simulink model "Control_model_10DOF_fin"  (R2016b)
settings: Solver=FixedStepAuto  StartTime=0.0  StopTime=10  FixedStep=0.0001  RelTol=1e-3
InitFcn:
  | Initialisation_ctr_10DOF_fin
values from neighbouring files (symbols this model uses):
  COM_Parameters = [-lpelvis/2;r2;0]    [Initialisation_ctr_10DOF_fin.m]
  DH_Parameters = [hfoot 0 ... (first row only)    [Initialisation_ctr_10DOF_fin.m]
  dTrunk = trunklbd(3)    [Initialisation_ctr_10DOF_fin.m]
  dxFootSM = dxFoot    [Initialisation_ctr_10DOF_fin.m]
  dxTrunk = 0.1    [Initialisation_ctr_10DOF_fin.m]
  Foot_Parameters = [0;-(lFoot/2-lHeel);0]    [Initialisation_ctr_10DOF_fin.m]
  HAA2HEE = [0; 0; 0.001]    [Initialisation_ctr_10DOF_fin.m]
  HEE2HFE = 0.5*[0.2; 0; 0]    [Initialisation_ctr_10DOF_fin.m]
  height_vrp = CoM_position(1)    [Initialisation_ctr_10DOF_fin.m]
  hTrunk = trunklbd(1)    [Initialisation_ctr_10DOF_fin.m]
  initial_CoM_position = R*CoM_position    [Initialisation_ctr_10DOF_fin.m]
  initial_CoM_velocity = [0;0;0]    [Initialisation_ctr_10DOF_fin.m]
  initial_left_foot = [0;0;-stance_width/2]    [Initialisation_ctr_10DOF_fin.m]
  initial_right_foot = [0;0;stance_width/2]    [Initialisation_ctr_10DOF_fin.m]
  initial_RorL = 0    [Initialisation_ctr_10DOF_fin.m]
  jointsinitial = [9;-15;6;0;0;6;-15;9]/180*pi    [Initialisation_ctr_10DOF_fin.m]
  K_DCM = 4.3*[1 0 0 ... (first row only)    [Initialisation_ctr_10DOF_fin.m]
  kD_left = mbody*[0.95 0 0 0 ... (first row only)    [Initialisation_ctr_10DOF_fin.m]
  kD_right = mbody*[0.12 0 0 0 ... (first row only)    [Initialisation_ctr_10DOF_fin.m]
  kI_left = mbody*[35 0 0 0 ... (first row only)    [Initialisation_ctr_10DOF_fin.m]
  kI_right = mbody*[38.2 0 0 0 ... (first row only)    [Initialisation_ctr_10DOF_fin.m]
  kP_left = mbody*[75 0 0 0 ... (first row only)    [Initialisation_ctr_10DOF_fin.m]
  kP_right = mbody*[5.6 0 0 0 ... (first row only)    [Initialisation_ctr_10DOF_fin.m]
  Lenght = [lShank;lThigh]    [Initialisation_ctr_10DOF_fin.m]
  lFootSM = lFoot    [Initialisation_ctr_10DOF_fin.m]
  lpelvis = wPelvis    [Initialisation_ctr_10DOF_fin.m]
  mass = mbody    (= 60)    [Initialisation_ctr_10DOF_fin.m]
  Masses = [mThigh; mShank; mTrunk]    [Initialisation_ctr_10DOF_fin.m]
  nb_step = 4    [Initialisation_ctr_10DOF_fin.m]
  nb_step_pattern = 20    [Initialisation_ctr_10DOF_fin.m]
  Pelvis_Parameters = [-lpelvis/2;hTrunk/2;0]    [Initialisation_ctr_10DOF_fin.m]
  stance_width = lpelvis    [Initialisation_ctr_10DOF_fin.m]
  stride_lenght = 0.50    (= 0.5)    [Initialisation_ctr_10DOF_fin.m]
  T_DS = time_DS    (= 0.4)    [Initialisation_ctr_10DOF_fin.m]
  T_IT = time_DS    (= 0.4)    [Initialisation_ctr_10DOF_fin.m]
  T_SS = time_swing    (= 1.6)    [Initialisation_ctr_10DOF_fin.m]
  time_DS = (time_stance-time_swing)/2    (= 0.4)    [Initialisation_ctr_10DOF_fin.m]
  time_stance = 60/100*time_stride    (= 2.4)    [Initialisation_ctr_10DOF_fin.m]
  time_step = time_stride/2    (= 2)    [Initialisation_ctr_10DOF_fin.m]
  time_swing = 40/100*time_stride    (= 1.6)    [Initialisation_ctr_10DOF_fin.m]
  validity_angle = [-20*pi/180 20*pi/180 ... (first row only)    [Initialisation_ctr_10DOF_fin.m]
  wTrunk = trunklbd(2)    [Initialisation_ctr_10DOF_fin.m]
  x4CoM = CoM_position(1)-XR4(1)    [Initialisation_ctr_10DOF_fin.m]
undefined symbols (not defined in the file or in its folder): dsegment, hFoot, l, lFoot, omega0_x, omega0_z, rho, wPelvis, X, Xp_x, Xp_z, Y, Z
undefined symbols (not defined in the file): k_grf, lShankSM, lThighSM, mShank, mThigh
libraries: nesl_utility x247, sm_lib x215, dspindex x12, FootPlacementLibrary x8, dspsigops x4, dspswit3 x1
(part 10 of 18)

== system Control_model_10DOF_fin/10DoF Walker SimMechanics Model/Graphic/Subsystem/Subsystem6 ==
  In1 : Inport
  Cartesian Joint : sm_lib/Joints/Cartesian Joint  SenseConstraintForce=off  SenseConstraintForceX=off  SenseConstraintForceY=off  SenseConstraintForceZ=off  SenseConstraintTorque=off  SenseConstraintTorqueX=off  SenseConstraintTorqueY=off  SenseConstraintTorqueZ=off  SenseTotalForce=off  SenseTotalForceX=off  SenseTotalForceY=off  SenseTotalForceZ=off  SenseTotalTorque=off  SenseTotalTorqueX=off  SenseTotalTorqueY=off  SenseTotalTorqueZ=off  CompositeWrenchDir=FollowerOnBase  CompositeWrenchFrame=BaseFrame  PxEquilibriumPosition=0  PxEquilibriumPositionUnits=m  PxSpringStiffness=0  PxSpringStiffnessUnits=N/m  PxDampingCoefficient=0  PxDampingCoefficientUnits=N/(m/s)  PxTorqueActuationMode=ComputedTorque  PxMotionActuationMode=InputMotion  PxSensePosition=off  PxSenseVelocity=off  PxSenseAcceleration=off  PxSenseTorqueForce=off  PxPositionTargetSpecify=on  PxPositionTargetPriority=Low  PxPositionTargetValue=0  PxPositionTargetValueUnits=m  PxVelocityTargetSpecify=off  PxVelocityTargetPriority=High  PxVelocityTargetValue=0  PxVelocityTargetValueUnits=m/s  PyEquilibriumPosition=0  PyEquilibriumPositionUnits=m  PySpringStiffness=0  PySpringStiffnessUnits=N/m  PyDampingCoefficient=0  PyDampingCoefficientUnits=N/(m/s)  PyTorqueActuationMode=ComputedTorque  PyMotionActuationMode=InputMotion  PySensePosition=off  PySenseVelocity=off  PySenseAcceleration=off  PySenseTorqueForce=off  PyPositionTargetSpecify=on  PyPositionTargetPriority=Low  PyPositionTargetValue=0  PyPositionTargetValueUnits=m  PyVelocityTargetSpecify=off  PyVelocityTargetPriority=High  PyVelocityTargetValue=0  PyVelocityTargetValueUnits=m/s  PzEquilibriumPosition=0  PzEquilibriumPositionUnits=m  PzSpringStiffness=0  PzSpringStiffnessUnits=N/m  PzDampingCoefficient=0  PzDampingCoefficientUnits=N/(m/s)  PzTorqueActuationMode=ComputedTorque  PzMotionActuationMode=InputMotion  PzSensePosition=off  PzSenseVelocity=off  PzSenseAcceleration=off  PzSenseTorqueForce=off  PzPositionTargetSpecify=on  PzPositionTargetPriority=Low  PzPositionTargetValue=0  PzPositionTargetValueUnits=m  PzVelocityTargetSpecify=off  PzVelocityTargetPriority=High  PzVelocityTargetValue=0  PzVelocityTargetValueUnits=m/s
  Demux : Demux  Outputs=3
  Graphic : sm_lib/Body Elements/Graphic  GraphicType=Marker  MarkerShape=Sphere  MarkerSize=10  GraphicVisPropType=SimpleVisualProperties  GraphicDiffuseColor=[0.2 0.2 1.0]  GraphicSpecularColor=[0.5 0.5 0.5 1.0]  GraphicAmbientColor=[0.15 0.15 0.15 1.0]  GraphicEmissiveColor=[0.0 0.0 0.0 1.0]  GraphicShininess=75  GraphicOpacity=1.0
  Memory2 : Memory  X0=[0;0;0]
  Rigid Transform1 : sm_lib/Frames and Transforms/Rigid Transform  TranslationMethod=None  TranslationStandardOffset=0  TranslationLengthUnit=m  TranslationStandardAxis=+Z  TranslationCartesianOffset=[0 0 0]  TranslationROffset=0  TranslationROffsetUnits=m  TranslationZOffset=0  TranslationZOffsetUnits=m  TranslationThetaOffset=0  TranslationThetaOffsetUnits=deg  RotationMethod=None  RotationAngleUnits=deg  RotationStandardAxis=+Z  RotationAngle=0.0  RotationArbitraryAxis=[0 0 1]  FollAlignAxisA=+X  BaseAlignAxisA=+Y  FollAlignAxisB=+Y  BaseAlignAxisB=+Z  RotationSequenceAxes=FollowerAxes  RotationSequence=XYX  RotationSequenceAngles=[0 0 0]  RotationSequenceAnglesUnits=deg  RotationMatrix=[1 0 0; 0 1 0; 0 0 1]
  Simulink-PS Converter1 : nesl_utility/Simulink-PS Converter  PhysicalDomain=network_engine_domain  SubClassName=ps_input  LeftPortType=input  RightPortType=output  PseudoPeriodic=off  Frequencies=[]  NoiseDistribution=none  NoiseParameters=[]  Unit=m  AffineConversion=on  InputFiltering=off  SimscapeFilterOrder=1  InputFilterTimeConstant=0.001  UdotUserProvided=1
  Simulink-PS Converter2 : nesl_utility/Simulink-PS Converter  PhysicalDomain=network_engine_domain  SubClassName=ps_input  LeftPortType=input  RightPortType=output  PseudoPeriodic=off  Frequencies=[]  NoiseDistribution=none  NoiseParameters=[]  Unit=m  AffineConversion=on  InputFiltering=off  SimscapeFilterOrder=1  InputFilterTimeConstant=0.001  UdotUserProvided=1
  Simulink-PS Converter7 : nesl_utility/Simulink-PS Converter  PhysicalDomain=network_engine_domain  SubClassName=ps_input  LeftPortType=input  RightPortType=output  PseudoPeriodic=off  Frequencies=[]  NoiseDistribution=none  NoiseParameters=[]  Unit=m  AffineConversion=on  InputFiltering=off  SimscapeFilterOrder=1  InputFilterTimeConstant=0.001  UdotUserProvided=1
  Conn1 : PMIOPort  Port=1  Side=Left
  wires:
  Demux/2 -> Simulink-PS Converter1/1
  Demux/3 -> Simulink-PS Converter2/1
  Demux/1 -> Simulink-PS Converter7/1
  In1/1 -> Memory2/1
  Memory2/1 -> Demux/1
  connections:
  Cartesian Joint/LConn1 -- Conn1/RConn1
  Simulink-PS Converter7/RConn1 -- Cartesian Joint/LConn2
  Simulink-PS Converter1/RConn1 -- Cartesian Joint/LConn3
  Simulink-PS Converter2/RConn1 -- Cartesian Joint/LConn4
  Rigid Transform1/LConn1 -- Cartesian Joint/RConn1
  Rigid Transform1/RConn1 -- Graphic/RConn1

== system Control_model_10DOF_fin/10DoF Walker SimMechanics Model/Graphic/Subsystem/Subsystem7 ==
  In1 : Inport
  Cartesian Joint : sm_lib/Joints/Cartesian Joint  SenseConstraintForce=off  SenseConstraintForceX=off  SenseConstraintForceY=off  SenseConstraintForceZ=off  SenseConstraintTorque=off  SenseConstraintTorqueX=off  SenseConstraintTorqueY=off  SenseConstraintTorqueZ=off  SenseTotalForce=off  SenseTotalForceX=off  SenseTotalForceY=off  SenseTotalForceZ=off  SenseTotalTorque=off  SenseTotalTorqueX=off  SenseTotalTorqueY=off  SenseTotalTorqueZ=off  CompositeWrenchDir=FollowerOnBase  CompositeWrenchFrame=BaseFrame  PxEquilibriumPosition=0  PxEquilibriumPositionUnits=m  PxSpringStiffness=0  PxSpringStiffnessUnits=N/m  PxDampingCoefficient=0  PxDampingCoefficientUnits=N/(m/s)  PxTorqueActuationMode=ComputedTorque  PxMotionActuationMode=InputMotion  PxSensePosition=off  PxSenseVelocity=off  PxSenseAcceleration=off  PxSenseTorqueForce=off  PxPositionTargetSpecify=on  PxPositionTargetPriority=Low  PxPositionTargetValue=0  PxPositionTargetValueUnits=m  PxVelocityTargetSpecify=off  PxVelocityTargetPriority=High  PxVelocityTargetValue=0  PxVelocityTargetValueUnits=m/s  PyEquilibriumPosition=0  PyEquilibriumPositionUnits=m  PySpringStiffness=0  PySpringStiffnessUnits=N/m  PyDampingCoefficient=0  PyDampingCoefficientUnits=N/(m/s)  PyTorqueActuationMode=ComputedTorque  PyMotionActuationMode=InputMotion  PySensePosition=off  PySenseVelocity=off  PySenseAcceleration=off  PySenseTorqueForce=off  PyPositionTargetSpecify=on  PyPositionTargetPriority=Low  PyPositionTargetValue=0  PyPositionTargetValueUnits=m  PyVelocityTargetSpecify=off  PyVelocityTargetPriority=High  PyVelocityTargetValue=0  PyVelocityTargetValueUnits=m/s  PzEquilibriumPosition=0  PzEquilibriumPositionUnits=m  PzSpringStiffness=0  PzSpringStiffnessUnits=N/m  PzDampingCoefficient=0  PzDampingCoefficientUnits=N/(m/s)  PzTorqueActuationMode=ComputedTorque  PzMotionActuationMode=InputMotion  PzSensePosition=off  PzSenseVelocity=off  PzSenseAcceleration=off  PzSenseTorqueForce=off  PzPositionTargetSpecify=on  PzPositionTargetPriority=Low  PzPositionTargetValue=0  PzPositionTargetValueUnits=m  PzVelocityTargetSpecify=off  PzVelocityTargetPriority=High  PzVelocityTargetValue=0  PzVelocityTargetValueUnits=m/s
  Demux : Demux  Outputs=3
  Graphic : sm_lib/Body Elements/Graphic  GraphicType=Marker  MarkerShape=Sphere  MarkerSize=10  GraphicVisPropType=SimpleVisualProperties  GraphicDiffuseColor=[0.2 0.2 1.0]  GraphicSpecularColor=[0.5 0.5 0.5 1.0]  GraphicAmbientColor=[0.15 0.15 0.15 1.0]  GraphicEmissiveColor=[0.0 0.0 0.0 1.0]  GraphicShininess=75  GraphicOpacity=1.0
  Memory2 : Memory  X0=[0;0;0]
  Rigid Transform1 : sm_lib/Frames and Transforms/Rigid Transform  TranslationMethod=None  TranslationStandardOffset=0  TranslationLengthUnit=m  TranslationStandardAxis=+Z  TranslationCartesianOffset=[0 0 0]  TranslationROffset=0  TranslationROffsetUnits=m  TranslationZOffset=0  TranslationZOffsetUnits=m  TranslationThetaOffset=0  TranslationThetaOffsetUnits=deg  RotationMethod=None  RotationAngleUnits=deg  RotationStandardAxis=+Z  RotationAngle=0.0  RotationArbitraryAxis=[0 0 1]  FollAlignAxisA=+X  BaseAlignAxisA=+Y  FollAlignAxisB=+Y  BaseAlignAxisB=+Z  RotationSequenceAxes=FollowerAxes  RotationSequence=XYX  RotationSequenceAngles=[0 0 0]  RotationSequenceAnglesUnits=deg  RotationMatrix=[1 0 0; 0 1 0; 0 0 1]
  Simulink-PS Converter1 : nesl_utility/Simulink-PS Converter  PhysicalDomain=network_engine_domain  SubClassName=ps_input  LeftPortType=input  RightPortType=output  PseudoPeriodic=off  Frequencies=[]  NoiseDistribution=none  NoiseParameters=[]  Unit=m  AffineConversion=on  InputFiltering=off  SimscapeFilterOrder=1  InputFilterTimeConstant=0.001  UdotUserProvided=1
  Simulink-PS Converter2 : nesl_utility/Simulink-PS Converter  PhysicalDomain=network_engine_domain  SubClassName=ps_input  LeftPortType=input  RightPortType=output  PseudoPeriodic=off  Frequencies=[]  NoiseDistribution=none  NoiseParameters=[]  Unit=m  AffineConversion=on  InputFiltering=off  SimscapeFilterOrder=1  InputFilterTimeConstant=0.001  UdotUserProvided=1
  Simulink-PS Converter7 : nesl_utility/Simulink-PS Converter  PhysicalDomain=network_engine_domain  SubClassName=ps_input  LeftPortType=input  RightPortType=output  PseudoPeriodic=off  Frequencies=[]  NoiseDistribution=none  NoiseParameters=[]  Unit=m  AffineConversion=on  InputFiltering=off  SimscapeFilterOrder=1  InputFilterTimeConstant=0.001  UdotUserProvided=1
  Conn1 : PMIOPort  Port=1  Side=Left
  wires:
  Demux/2 -> Simulink-PS Converter1/1
  Demux/3 -> Simulink-PS Converter2/1
  Demux/1 -> Simulink-PS Converter7/1
  In1/1 -> Memory2/1
  Memory2/1 -> Demux/1
  connections:
  Cartesian Joint/LConn1 -- Conn1/RConn1
  Simulink-PS Converter7/RConn1 -- Cartesian Joint/LConn2
  Simulink-PS Converter1/RConn1 -- Cartesian Joint/LConn3
  Simulink-PS Converter2/RConn1 -- Cartesian Joint/LConn4
  Rigid Transform1/LConn1 -- Cartesian Joint/RConn1
  Rigid Transform1/RConn1 -- Graphic/RConn1

== system Control_model_10DOF_fin/10DoF Walker SimMechanics Model/Graphic/Subsystem/Subsystem8 ==
  In1 : Inport
  Cartesian Joint : sm_lib/Joints/Cartesian Joint  SenseConstraintForce=off  SenseConstraintForceX=off  SenseConstraintForceY=off  SenseConstraintForceZ=off  SenseConstraintTorque=off  SenseConstraintTorqueX=off  SenseConstraintTorqueY=off  SenseConstraintTorqueZ=off  SenseTotalForce=off  SenseTotalForceX=off  SenseTotalForceY=off  SenseTotalForceZ=off  SenseTotalTorque=off  SenseTotalTorqueX=off  SenseTotalTorqueY=off  SenseTotalTorqueZ=off  CompositeWrenchDir=FollowerOnBase  CompositeWrenchFrame=BaseFrame  PxEquilibriumPosition=0  PxEquilibriumPositionUnits=m  PxSpringStiffness=0  PxSpringStiffnessUnits=N/m  PxDampingCoefficient=0  PxDampingCoefficientUnits=N/(m/s)  PxTorqueActuationMode=ComputedTorque  PxMotionActuationMode=InputMotion  PxSensePosition=off  PxSenseVelocity=off  PxSenseAcceleration=off  PxSenseTorqueForce=off  PxPositionTargetSpecify=on  PxPositionTargetPriority=Low  PxPositionTargetValue=0  PxPositionTargetValueUnits=m  PxVelocityTargetSpecify=off  PxVelocityTargetPriority=High  PxVelocityTargetValue=0  PxVelocityTargetValueUnits=m/s  PyEquilibriumPosition=0  PyEquilibriumPositionUnits=m  PySpringStiffness=0  PySpringStiffnessUnits=N/m  PyDampingCoefficient=0  PyDampingCoefficientUnits=N/(m/s)  PyTorqueActuationMode=ComputedTorque  PyMotionActuationMode=InputMotion  PySensePosition=off  PySenseVelocity=off  PySenseAcceleration=off  PySenseTorqueForce=off  PyPositionTargetSpecify=on  PyPositionTargetPriority=Low  PyPositionTargetValue=0  PyPositionTargetValueUnits=m  PyVelocityTargetSpecify=off  PyVelocityTargetPriority=High  PyVelocityTargetValue=0  PyVelocityTargetValueUnits=m/s  PzEquilibriumPosition=0  PzEquilibriumPositionUnits=m  PzSpringStiffness=0  PzSpringStiffnessUnits=N/m  PzDampingCoefficient=0  PzDampingCoefficientUnits=N/(m/s)  PzTorqueActuationMode=ComputedTorque  PzMotionActuationMode=InputMotion  PzSensePosition=off  PzSenseVelocity=off  PzSenseAcceleration=off  PzSenseTorqueForce=off  PzPositionTargetSpecify=on  PzPositionTargetPriority=Low  PzPositionTargetValue=0  PzPositionTargetValueUnits=m  PzVelocityTargetSpecify=off  PzVelocityTargetPriority=High  PzVelocityTargetValue=0  PzVelocityTargetValueUnits=m/s
  Demux : Demux  Outputs=3
  Graphic : sm_lib/Body Elements/Graphic  GraphicType=Marker  MarkerShape=Sphere  MarkerSize=15  GraphicVisPropType=SimpleVisualProperties  GraphicDiffuseColor=[1.0 0.8 0.8]  GraphicSpecularColor=[0.5 0.5 0.5 1.0]  GraphicAmbientColor=[0.15 0.15 0.15 1.0]  GraphicEmissiveColor=[0.0 0.0 0.0 1.0]  GraphicShininess=75  GraphicOpacity=1.0
  Memory2 : Memory  X0=[0;0;0]
  Rigid Transform1 : sm_lib/Frames and Transforms/Rigid Transform  TranslationMethod=None  TranslationStandardOffset=0  TranslationLengthUnit=m  TranslationStandardAxis=+Z  TranslationCartesianOffset=[0 0 0]  TranslationROffset=0  TranslationROffsetUnits=m  TranslationZOffset=0  TranslationZOffsetUnits=m  TranslationThetaOffset=0  TranslationThetaOffsetUnits=deg  RotationMethod=None  RotationAngleUnits=deg  RotationStandardAxis=+Z  RotationAngle=0.0  RotationArbitraryAxis=[0 0 1]  FollAlignAxisA=+X  BaseAlignAxisA=+Y  FollAlignAxisB=+Y  BaseAlignAxisB=+Z  RotationSequenceAxes=FollowerAxes  RotationSequence=XYX  RotationSequenceAngles=[0 0 0]  RotationSequenceAnglesUnits=deg  RotationMatrix=[1 0 0; 0 1 0; 0 0 1]
  Simulink-PS Converter1 : nesl_utility/Simulink-PS Converter  PhysicalDomain=network_engine_domain  SubClassName=ps_input  LeftPortType=input  RightPortType=output  PseudoPeriodic=off  Frequencies=[]  NoiseDistribution=none  NoiseParameters=[]  Unit=m  AffineConversion=on  InputFiltering=off  SimscapeFilterOrder=1  InputFilterTimeConstant=0.001  UdotUserProvided=1
  Simulink-PS Converter2 : nesl_utility/Simulink-PS Converter  PhysicalDomain=network_engine_domain  SubClassName=ps_input  LeftPortType=input  RightPortType=output  PseudoPeriodic=off  Frequencies=[]  NoiseDistribution=none  NoiseParameters=[]  Unit=m  AffineConversion=on  InputFiltering=off  SimscapeFilterOrder=1  InputFilterTimeConstant=0.001  UdotUserProvided=1
  Simulink-PS Converter7 : nesl_utility/Simulink-PS Converter  PhysicalDomain=network_engine_domain  SubClassName=ps_input  LeftPortType=input  RightPortType=output  PseudoPeriodic=off  Frequencies=[]  NoiseDistribution=none  NoiseParameters=[]  Unit=m  AffineConversion=on  InputFiltering=off  SimscapeFilterOrder=1  InputFilterTimeConstant=0.001  UdotUserProvided=1
  Conn1 : PMIOPort  Port=1  Side=Left
  wires:
  Demux/2 -> Simulink-PS Converter1/1
  Demux/3 -> Simulink-PS Converter2/1
  Demux/1 -> Simulink-PS Converter7/1
  In1/1 -> Memory2/1
  Memory2/1 -> Demux/1
  connections:
  Cartesian Joint/LConn1 -- Conn1/RConn1
  Simulink-PS Converter7/RConn1 -- Cartesian Joint/LConn2
  Simulink-PS Converter1/RConn1 -- Cartesian Joint/LConn3
  Simulink-PS Converter2/RConn1 -- Cartesian Joint/LConn4
  Rigid Transform1/LConn1 -- Cartesian Joint/RConn1
  Rigid Transform1/RConn1 -- Graphic/RConn1

== system Control_model_10DOF_fin/Control/Double_Support/Left stance phase1/Stance leg position_initial ==
  position : Inport  PortDimensions=4
  velocity : Inport  Port=2  PortDimensions=4
  theta4 : Inport  Port=3
  Constant : Constant  Value=jointsinitial(1:4)
  Demux : Demux
  Mux : Mux
  PID right : Subsystem
  Scope x1 : Subsystem
  Sum1 : Sum  Inputs=-+|
  Terminator : Terminator
  torques : Outport
  wires:
  PID right/1(torques_des) -> torques/1
  position/1 -> Sum1/1
  Sum1/1 -> Scope x1/1(Input), PID right/1(error)
  velocity/1 -> PID right/2(velocity)
  Constant/1 -> Demux/1
  Mux/1 -> Sum1/2
  Demux/1 -> Mux/1
  Demux/3 -> Mux/3
  Demux/2 -> Mux/2
  theta4/1 -> Mux/4
  Demux/4 -> Terminator/1

== system Control_model_10DOF_fin/Control/Double_Support/Left stance phase1/Stance leg position_initial1 ==
  position : Inport  PortDimensions=4
  velocity : Inport  Port=2  PortDimensions=4
  theta5 : Inport  Port=3
  knee_trajectory : Inport  Port=4
  Constant : Constant  Value=jointsinitial(5:8)
  Demux1 : Demux
  Mux1 : Mux
  PID left : Subsystem
  Scope : Scope
  Scope x2 : Subsystem
  Sum1 : Sum  Inputs=-+|
  Terminator : Terminator
  Terminator1 : Terminator
  torques : Outport
  wires:
  position/1 -> Scope x2/1(Input), Sum1/1
  Sum1/1 -> Scope/1, PID left/1(error)
  velocity/1 -> PID left/2(velocity)
  PID left/1(torques_des) -> torques/1
  Constant/1 -> Demux1/1
  Mux1/1 -> Scope x2/2(Input1), Sum1/2
  Demux1/2 -> Mux1/2
  Demux1/4 -> Mux1/4
  theta5/1 -> Mux1/1
  knee_trajectory/1 -> Mux1/3
  Demux1/1 -> Terminator/1
  Demux1/3 -> Terminator1/1

== system Control_model_10DOF_fin/Control/Double_Support/Left stance phase1/Subsystem ==
  DCM_position : Inport
  DCM_velocity : Inport  Port=2
  FK_info : Inport  Port=3
  Bus Selector : BusSelector  OutputSignals=XWcom,VWcom
  Bus Selector1 : BusSelector  OutputSignals=JRcom,JLcom,TWR,TWL
  Bus Selector3 : BusSelector  OutputSignals=TWR,TWL
  Bus Selector4 : BusSelector  OutputSignals=XWcom
  MATLAB Function1 : MATLAB Function  TreatAsAtomicUnit=on
  MATLAB Function2 : MATLAB Function  TreatAsAtomicUnit=on
  MATLAB Function3 : MATLAB Function  TreatAsAtomicUnit=on
  MATLAB Function4 : MATLAB Function  TreatAsAtomicUnit=on
  MATLAB Function5 : MATLAB Function  TreatAsAtomicUnit=on
  Scope1 : Scope
  Terminator : Terminator
  Terminator1 : Terminator
  Terminator2 : Terminator
  VRP based DCM tracking control : MATLAB Function  TreatAsAtomicUnit=on
  extrapolated CoM calcul : MATLAB Function  TreatAsAtomicUnit=on
  Torques_des : Outport  OutDataTypeStr=double  Unit=N*m
  Force_des : Outport  Port=2
  r_vrp : Outport  Port=3
  r_extrapolated_CoM : Outport  Port=4
  wires:
  DCM_position/1 -> VRP based DCM tracking control/3(DCM_position)
  extrapolated CoM calcul/1(r_extrapolate_CoM) -> r_extrapolated_CoM/1, VRP based DCM tracking control/1(r_extrapolated_CoM)
  DCM_velocity/1 -> VRP based DCM tracking control/2(DCM_velocity)
  FK_info/1 -> Bus Selector/1, Bus Selector3/1, Bus Selector4/1, Bus Selector1/1
  VRP based DCM tracking control/1(r_vrp) -> MATLAB Function4/1(r_vrp), MATLAB Function5/1(r_vrp_W), MATLAB Function1/1(r_vrp_W)
  Bus Selector/1 -> extrapolated CoM calcul/1(CoM_position)  "<XWcom>"
  Bus Selector/2 -> extrapolated CoM calcul/2(CoM_velocity)  "<VWcom>"
  Bus Selector4/1 -> MATLAB Function4/2(r_CoM), MATLAB Function2/2(r_CoM)  "<XWcom>"
  Bus Selector3/2 -> MATLAB Function1/3(TWL)  "<TWL>"
  MATLAB Function3/1(Torques_des) -> Torques_des/1
  MATLAB Function3/2(alpha) -> Scope1/1
  Bus Selector1/4 -> MATLAB Function3/6(TWL)  "<TWL>"
  Bus Selector1/3 -> MATLAB Function3/5(TWR)  "<TWR>"
  Bus Selector1/2 -> MATLAB Function3/4(JcomL)  "<JLcom>"
  Bus Selector1/1 -> MATLAB Function3/3(JcomR)  "<JRcom>"
  MATLAB Function2/1(Force_des) -> MATLAB Function3/1(Force_des)
  Bus Selector3/1 -> MATLAB Function4/3(TWR), MATLAB Function5/2(TWR), MATLAB Function1/2(TWR)  "<TWR>"
  MATLAB Function1/2(alpha) -> MATLAB Function3/2("alpha ")
  MATLAB Function5/1(new_vrp_W) -> MATLAB Function2/1(r_vrp), r_vrp/1
  MATLAB Function4/1(Force_des) -> Force_des/1
  MATLAB Function1/1(new_vrp_W) -> Terminator/1
  MATLAB Function5/3(cas) -> Terminator1/1
  MATLAB Function5/2(outside) -> Terminator2/1

== system Control_model_10DOF_fin/Control/Double_Support/Right stance phase/Stance leg position_initial ==
  position : Inport  PortDimensions=4
  velocity : Inport  Port=2  PortDimensions=4
  theta4 : Inport  Port=3
  knee_trajectory : Inport  Port=4
  Constant : Constant  Value=jointsinitial(1:4)
  Demux : Demux
  Mux : Mux
  PID right : Subsystem
  Scope x2 : Subsystem
  Sum1 : Sum  Inputs=-+|
  Terminator : Terminator
  Terminator1 : Terminator
  torques : Outport
  wires:
  PID right/1(torques_des) -> torques/1
  position/1 -> Scope x2/1(Input), Sum1/1
  Sum1/1 -> PID right/1(error)
  velocity/1 -> PID right/2(velocity)
  Constant/1 -> Demux/1
  Mux/1 -> Scope x2/2(Input1), Sum1/2
  Demux/1 -> Mux/1
  Demux/3 -> Mux/3
  theta4/1 -> Mux/4
  knee_trajectory/1 -> Mux/2
  Demux/2 -> Terminator/1
  Demux/4 -> Terminator1/1

== system Control_model_10DOF_fin/Control/Double_Support/Right stance phase/Stance leg position_initial1 ==
  position : Inport  PortDimensions=4
  velocity : Inport  Port=2  PortDimensions=4
  theta5 : Inport  Port=3
  Constant : Constant  Value=jointsinitial(5:8)
  Demux1 : Demux
  Mux1 : Mux
  PID left : Subsystem
  Scope x2 : Subsystem
  Sum1 : Sum  Inputs=-+|
  Terminator : Terminator
  torques : Outport
  wires:
  position/1 -> Scope x2/1(Input), Sum1/1
  Sum1/1 -> PID left/1(error)
  velocity/1 -> PID left/2(velocity)
  PID left/1(torques_des) -> torques/1
  Constant/1 -> Demux1/1
  Mux1/1 -> Scope x2/2(Input1), Sum1/2
  Demux1/2 -> Mux1/2
  Demux1/3 -> Mux1/3
  Demux1/4 -> Mux1/4
  theta5/1 -> Mux1/1
  Demux1/1 -> Terminator/1

== system Control_model_10DOF_fin/Control/Double_Support/Right stance phase/Subsystem ==
  DCM_position : Inport
  DCM_velocity : Inport  Port=2
  FK_info : Inport  Port=3
  Bus Selector : BusSelector  OutputSignals=XWcom,VWcom
  Bus Selector1 : BusSelector  OutputSignals=JRcom,JLcom,TWR,TWL
  Bus Selector3 : BusSelector  OutputSignals=TWR,TWL
  Bus Selector4 : BusSelector  OutputSignals=XWcom
  MATLAB Function : MATLAB Function  TreatAsAtomicUnit=on
  MATLAB Function1 : MATLAB Function  TreatAsAtomicUnit=on
  MATLAB Function2 : MATLAB Function  TreatAsAtomicUnit=on
  MATLAB Function3 : MATLAB Function  TreatAsAtomicUnit=on
  MATLAB Function5 : MATLAB Function  TreatAsAtomicUnit=on
  Scope1 : Scope
  Terminator{,1..3} (4 alike) : Terminator
  VRP based DCM tracking control : MATLAB Function  TreatAsAtomicUnit=on
  extrapolated CoM calcul : MATLAB Function  TreatAsAtomicUnit=on
  Torques_des : Outport  OutDataTypeStr=double  Unit=N*m
  Force_des : Outport  Port=2
  r_vrp : Outport  Port=3
  r_extrapolated_CoM : Outport  Port=4
  wires:
  Bus Selector1/1 -> MATLAB Function3/3(JcomR)  "<JRcom>"
  DCM_position/1 -> VRP based DCM tracking control/3(DCM_position)
  MATLAB Function3/1(Torques_des) -> Torques_des/1
  MATLAB Function/1(Force_des) -> MATLAB Function3/1(Force_des)
  extrapolated CoM calcul/1(r_extrapolate_CoM) -> r_extrapolated_CoM/1, VRP based DCM tracking control/1(r_extrapolated_CoM)
  DCM_velocity/1 -> VRP based DCM tracking control/2(DCM_velocity)
  FK_info/1 -> Bus Selector/1, Bus Selector1/1, Bus Selector4/1, Bus Selector3/1
  MATLAB Function3/2(alpha) -> Scope1/1
  Bus Selector/1 -> extrapolated CoM calcul/1(CoM_position)  "<XWcom>"
  Bus Selector/2 -> extrapolated CoM calcul/2(CoM_velocity)  "<VWcom>"
  Bus Selector3/1 -> MATLAB Function5/2(TWR)  "<TWR>"
  Bus Selector4/1 -> MATLAB Function2/2(r_CoM), MATLAB Function/2(r_CoM)  "<XWcom>"
  Bus Selector3/2 -> MATLAB Function2/3(TWL), MATLAB Function1/2(TWL), MATLAB Function5/3(TWL)  "<TWL>"
  Bus Selector1/2 -> MATLAB Function3/4(JcomL)  "<JLcom>"
  Bus Selector1/3 -> MATLAB Function3/5(TWR)  "<TWR>"
  Bus Selector1/4 -> MATLAB Function3/6(TWL)  "<TWL>"
  MATLAB Function5/2(alpha) -> MATLAB Function3/2("alpha ")
  MATLAB Function1/1(new_vrp_W) -> MATLAB Function/1(r_vrp)
  VRP based DCM tracking control/1(r_vrp) -> MATLAB Function2/1(r_vrp), MATLAB Function1/1(r_vrp_W), r_vrp/1, MATLAB Function5/1(r_vrp_W)
  MATLAB Function2/1(Force_des) -> Force_des/1
  MATLAB Function5/3(cas) -> Terminator/1
  MATLAB Function1/2(outside) -> Terminator1/1
  MATLAB Function1/3(cas) -> Terminator2/1
  MATLAB Function5/1(new_vrp_W) -> Terminator3/1

== system Control_model_10DOF_fin/Control/Finish_Swing_Phase/Left Swing // Right Stance/Left Swing leg control ==
  swing_state : Inport
  actual_joint_angle : Inport  Port=2
  FK_info : Inport  Port=3
  actual_joint_velocity : Inport  Port=4
  theta7 : Inport  Port=5
  Bus Selector : BusSelector  OutputSignals=TR5,TR8,TR9,TRL,TWR
  Left : MATLAB Function  TreatAsAtomicUnit=on
  PID left : Subsystem
  Saturation : Saturate  UpperLimit=validity_angle(5:8,2)  LowerLimit=validity_angle(5:8,1)
  Scope : Scope
  Scope x1 : Subsystem
  Scope x2 : Subsystem
  Sum : Sum  Inputs=-+|
  Terminator : Terminator
  Torques_des : Outport  OutDataTypeStr=double  Unit=N*m  PortDimensions=4
  wires:
  Left/1(desired_joint_angle) -> Saturation/1
  Sum/1 -> PID left/1(error)
  actual_joint_angle/1 -> Left/8(actual_joint_angle), Scope x2/1(Input), Sum/1
  FK_info/1 -> Bus Selector/1
  actual_joint_velocity/1 -> PID left/2(velocity)
  PID left/1(torques_des) -> Torques_des/1
  swing_state/1 -> Scope x1/1(Input), Left/6(swing_state)
  Bus Selector/3 -> Left/3(TR9)  "<TR9>"
  Bus Selector/4 -> Left/4(TRL)  "<TRL>"
  Bus Selector/1 -> Left/1(TR5)  "<TR5>"
  Saturation/1 -> Sum/2, Scope x2/2(Input1)
  Bus Selector/2 -> Left/2(TR8)  "<TR8>"
  Bus Selector/5 -> Left/5(TWR)  "<TWR>"
  Left/3(cas) -> Scope/1
  theta7/1 -> Left/7(desired_knee_angle)
  Left/2(ok) -> Terminator/1

== system Control_model_10DOF_fin/Control/Finish_Swing_Phase/Left Swing // Right Stance/Martijn Step adjustement ==
  FK_info : Inport
  R_or_L : Inport  Port=2
  Bus Selector : BusSelector  OutputSignals=XWcom,VWcom
  Constant1 : Constant  Value=time_swing
  Terminator : Terminator
  xCoM pred : Subsystem
  StepPos : Outport
  wires:
  Constant1/1 -> xCoM pred/1(T)
  R_or_L/1 -> xCoM pred/4(R_or_L)
  FK_info/1 -> Bus Selector/1
  Bus Selector/2 -> xCoM pred/3(Vcom)  "<VWcom>"
  Bus Selector/1 -> xCoM pred/2(Xcom)  "<XWcom>"
  xCoM pred/1(StepPos) -> StepPos/1
  xCoM pred/2(xCoMpred) -> Terminator/1

== system Control_model_10DOF_fin/Control/Finish_Swing_Phase/Left Swing // Right Stance/Right Stance leg control ==
  DCM_position : Inport
  DCM_velocity : Inport  Port=2
  FK_info : Inport  Port=3
  Bus Selector : BusSelector  OutputSignals=XWcom,VWcom
  Bus Selector1 : BusSelector  OutputSignals=JRcom,TWR
  Bus Selector3 : BusSelector  OutputSignals=TWR
  Bus Selector4 : BusSelector  OutputSignals=XWcom
  DCM calcul : MATLAB Function  TreatAsAtomicUnit=on
  MATLAB Function : MATLAB Function  TreatAsAtomicUnit=on
  MATLAB Function1 : MATLAB Function  TreatAsAtomicUnit=on
  MATLAB Function2 : MATLAB Function  TreatAsAtomicUnit=on
  MATLAB Function5 : MATLAB Function  TreatAsAtomicUnit=on
  Terminator : Terminator
  Terminator1 : Terminator
  VRP based DCM tracking control : MATLAB Function  TreatAsAtomicUnit=on
  Torques_des : Outport  OutDataTypeStr=double  Unit=N*m
  Force_des : Outport  Port=2
  r_vrp : Outport  Port=3
  r_extrapolated_CoM : Outport  Port=4
  wires:
  Bus Selector1/1 -> MATLAB Function1/2(JcomR)  "<JRcom>"
  MATLAB Function1/1(Torques_des) -> Torques_des/1
  DCM_position/1 -> VRP based DCM tracking control/3(DCM_position)
  MATLAB Function/1(Force_des) -> MATLAB Function1/1(Force_des_W)
  DCM_velocity/1 -> VRP based DCM tracking control/2(DCM_velocity)
  DCM calcul/1(r_extrapolated_CoM) -> VRP based DCM tracking control/1(r_extrapolated_CoM), r_extrapolated_CoM/1
  FK_info/1 -> Bus Selector/1, Bus Selector4/1, Bus Selector1/1, Bus Selector3/1
  Bus Selector/1 -> DCM calcul/1(CoM_position)  "<XWcom>"
  Bus Selector4/1 -> MATLAB Function2/2(r_CoM), MATLAB Function/2(r_CoM)  "<XWcom>"
  Bus Selector/2 -> DCM calcul/2(CoM_velocity)  "<VWcom>"
  Bus Selector3/1 -> MATLAB Function2/3(TWR), MATLAB Function5/2(TWR)  "<TWR>"
  VRP based DCM tracking control/1(r_vrp) -> MATLAB Function2/1(r_vrp), MATLAB Function5/1(r_vrp_W)
  MATLAB Function5/1(new_vrp_W) -> MATLAB Function/1(r_vrp), r_vrp/1
  Bus Selector1/2 -> MATLAB Function1/3(TWR)  "<TWR>"
  MATLAB Function2/1(Force_des) -> Force_des/1
  MATLAB Function5/2(outside) -> Terminator/1
  MATLAB Function5/3(cas) -> Terminator1/1

== system Control_model_10DOF_fin/Control/Finish_Swing_Phase/Left Swing // Right Stance/Scope x1 ==
  Input : Inport
  Demux : Demux  Outputs=3
  Scope1 : Scope
  Scope2 : Scope
  Scope3 : Scope
  wires:
  Input/1 -> Demux/1
  Demux/2 -> Scope1/1
  Demux/3 -> Scope2/1
  Demux/1 -> Scope3/1

== system Control_model_10DOF_fin/Control/Finish_Swing_Phase/Left Swing // Right Stance/Scope x8 ==
  Input : Inport
  Demux : Demux  Outputs=3
  Scope1 : Scope
  Scope2 : Scope
  Scope3 : Scope
  wires:
  Input/1 -> Demux/1
  Demux/2 -> Scope1/1
  Demux/3 -> Scope2/1
  Demux/1 -> Scope3/1

== system Control_model_10DOF_fin/Control/Finish_Swing_Phase/Left Swing // Right Stance/Stance leg position_initial ==
  position : Inport  PortDimensions=4
  velocity : Inport  Port=2  PortDimensions=4
  hip_trajectory : Inport  Port=3
  theta2 : Inport  Port=4
  Constant : Constant  Value=jointsinitial(1:4)
  Demux : Demux
  Mux : Mux
  PID right : Subsystem
  Scope x2 : Subsystem
  Sum1 : Sum  Inputs=-+|
  Terminator : Terminator
  Terminator1 : Terminator
  torques : Outport
  wires:
  PID right/1(torques_des) -> torques/1
  position/1 -> Scope x2/1(Input), Sum1/1
  Sum1/1 -> PID right/1(error)
  velocity/1 -> PID right/2(velocity)
  Constant/1 -> Demux/1
  Mux/1 -> Scope x2/2(Input1), Sum1/2
  Demux/1 -> Mux/1
  Demux/3 -> Mux/3
  hip_trajectory/1 -> Mux/4
  theta2/1 -> Mux/2
  Demux/2 -> Terminator/1
  Demux/4 -> Terminator1/1

== system Control_model_10DOF_fin/Control/Finish_Swing_Phase/Right Swing // Left Stance1/Martijn Step adjustement ==
  FK_info : Inport
  R_or_L : Inport  Port=2
  Bus Selector : BusSelector  OutputSignals=XWcom,VWcom
  Constant1 : Constant  Value=time_swing
  Terminator : Terminator
  xCoM pred : Subsystem
  StepPos : Outport
  wires:
  Constant1/1 -> xCoM pred/1(T)
  R_or_L/1 -> xCoM pred/4(R_or_L)
  FK_info/1 -> Bus Selector/1
  Bus Selector/2 -> xCoM pred/3(Vcom)  "<VWcom>"
  Bus Selector/1 -> xCoM pred/2(Xcom)  "<XWcom>"
  xCoM pred/1(StepPos) -> StepPos/1
  xCoM pred/2(xCoMpred) -> Terminator/1

== system Control_model_10DOF_fin/Control/Finish_Swing_Phase/Right Swing // Left Stance1/Right Swing leg control ==
  swing_state : Inport
  actual_joint_angle : Inport  Port=2
  FK_info : Inport  Port=3
  actual_joint_velocity : Inport  Port=4
  theta2 : Inport  Port=5
  Bus Selector : BusSelector  OutputSignals=TL4,TL1,TL0,TLR,TWL
  PID right : Subsystem
  Right : MATLAB Function  TreatAsAtomicUnit=on
  Saturation : Saturate  UpperLimit=validity_angle(1:4,2)  LowerLimit=validity_angle(1:4,1)
  Scope x2 : Subsystem
  Scope1 : Scope
  Scope2 : Scope
  Sum : Sum  Inputs=-+|
  Torques_des : Outport  OutDataTypeStr=double  Unit=N*m  PortDimensions=4
  wires:
  Right/1(desired_joint_angle) -> Saturation/1
  Sum/1 -> PID right/1(error)
  actual_joint_angle/1 -> Right/8(actual_joint_angle), Scope x2/1(Input), Sum/1
  FK_info/1 -> Bus Selector/1
  swing_state/1 -> Right/6(swing_state)
  actual_joint_velocity/1 -> PID right/2(velocity)
  PID right/1(torques_des) -> Torques_des/1
  Bus Selector/1 -> Right/1(TL4)  "<TL4>"
  Bus Selector/2 -> Right/2(TL1)  "<TL1>"
  Bus Selector/3 -> Right/3(TL0)  "<TL0>"
  Bus Selector/4 -> Right/4(TLR)  "<TLR>"
  Bus Selector/5 -> Right/5(TWL)  "<TWL>"
  Right/3(cas) -> Scope1/1
  Saturation/1 -> Sum/2, Scope x2/2(Input1)
  Right/2(ok) -> Scope2/1
  theta2/1 -> Right/7(desired_knee_angle)

== system Control_model_10DOF_fin/Control/Finish_Swing_Phase/Right Swing // Left Stance1/Stance leg control ==
  DCM_position : Inport
  DCM_velocity : Inport  Port=2
  FK_info : Inport  Port=3
  Bus Selector : BusSelector  OutputSignals=XWcom,VWcom
  Bus Selector1 : BusSelector  OutputSignals=JLcom,TWL
  Bus Selector2 : BusSelector  OutputSignals=TWL
  Bus Selector3 : BusSelector  OutputSignals=XWcom
  DCM calcul : MATLAB Function  TreatAsAtomicUnit=on
  MATLAB Function : MATLAB Function  TreatAsAtomicUnit=on
  MATLAB Function1 : MATLAB Function  TreatAsAtomicUnit=on
  MATLAB Function2 : MATLAB Function  TreatAsAtomicUnit=on
  MATLAB Function5 : MATLAB Function  TreatAsAtomicUnit=on
  Terminator : Terminator
  Terminator1 : Terminator
  VRP based DCM tracking control : MATLAB Function  TreatAsAtomicUnit=on
  Torques_des : Outport  OutDataTypeStr=double  Unit=N*m
  Force_des : Outport  Port=2
  r_vrp : Outport  Port=3
  r_extrapolated_CoM : Outport  Port=4
  wires:
  DCM_position/1 -> VRP based DCM tracking control/3(DCM_position)
  DCM_velocity/1 -> VRP based DCM tracking control/2(DCM_velocity)
  Bus Selector/1 -> DCM calcul/1(CoM_position)  "<XWcom>"
  DCM calcul/1(r_DCM) -> VRP based DCM tracking control/1(r_DCM), r_extrapolated_CoM/1
  MATLAB Function/1(Force_des) -> MATLAB Function2/1(Force_des)
  MATLAB Function2/1(Torques_des) -> Torques_des/1
  Bus Selector/2 -> DCM calcul/2(CoM_velocity)  "<VWcom>"
  Bus Selector1/1 -> MATLAB Function2/2(JcomL)  "<JLcom>"
  MATLAB Function5/1(new_vrp_W) -> MATLAB Function/1(r_vrp), r_vrp/1
  VRP based DCM tracking control/1(r_vrp) -> MATLAB Function1/1(r_vrp), MATLAB Function5/1(r_vrp_W)
  Bus Selector2/1 -> MATLAB Function1/3(TWL), MATLAB Function5/2(TWL)  "<TWL>"
  Bus Selector3/1 -> MATLAB Function1/2(r_CoM), MATLAB Function/2(r_CoM)  "<XWcom>"
  Bus Selector1/2 -> MATLAB Function2/3(TWL)  "<TWL>"
  FK_info/1 -> Bus Selector1/1, Bus Selector3/1, Bus Selector2/1, Bus Selector/1
  MATLAB Function1/1(Force_des) -> Force_des/1
  MATLAB Function5/2(outside) -> Terminator/1
  MATLAB Function5/3(cas) -> Terminator1/1

== system Control_model_10DOF_fin/Control/Finish_Swing_Phase/Right Swing // Left Stance1/Stance leg position_initial1 ==
  position : Inport  PortDimensions=4
  velocity : Inport  Port=2  PortDimensions=4
  hip_trajectory : Inport  Port=3
  theta7 : Inport  Port=4
  Constant : Constant  Value=jointsinitial(5:8)
  Demux1 : Demux
  Mux1 : Mux
  PID left : Subsystem
  Scope : Scope
  Sum1 : Sum  Inputs=-+|
  Terminator : Terminator
  Terminator1 : Terminator
  torques : Outport
  wires:
  position/1 -> Sum1/1
  Sum1/1 -> Scope/1, PID left/1(error)
  velocity/1 -> PID left/2(velocity)
  PID left/1(torques_des) -> torques/1
  Constant/1 -> Demux1/1
  Mux1/1 -> Sum1/2
  Demux1/2 -> Mux1/2
  Demux1/4 -> Mux1/4
  hip_trajectory/1 -> Mux1/1
  theta7/1 -> Mux1/3
  Demux1/1 -> Terminator/1
  Demux1/3 -> Terminator1/1

== system Control_model_10DOF_fin/Control/Inititial_Transfert/Left stance phase1/Stance leg position_initial ==
  position : Inport  PortDimensions=4
  velocity : Inport  Port=2  PortDimensions=4
  theta4 : Inport  Port=3
  Constant : Constant  Value=jointsinitial(1:4)
  Demux : Demux
  Mux : Mux
  PID right : Subsystem
  Scope x1 : Subsystem
  Sum1 : Sum  Inputs=-+|
  Terminator : Terminator
  torques : Outport
  wires:
  PID right/1(torques_des) -> torques/1
  position/1 -> Sum1/1
  Sum1/1 -> Scope x1/1(Input), PID right/1(error)
  velocity/1 -> PID right/2(velocity)
  Constant/1 -> Demux/1
  Mux/1 -> Sum1/2
  Demux/1 -> Mux/1
  Demux/3 -> Mux/3
  Demux/2 -> Mux/2
  theta4/1 -> Mux/4
  Demux/4 -> Terminator/1

== system Control_model_10DOF_fin/Control/Inititial_Transfert/Left stance phase1/Stance leg position_initial1 ==
  position : Inport  PortDimensions=4
  velocity : Inport  Port=2  PortDimensions=4
  theta5 : Inport  Port=3
  Constant : Constant  Value=jointsinitial(5:8)
  Demux1 : Demux
  Mux1 : Mux
  PID left : Subsystem
  Scope : Scope
  Sum1 : Sum  Inputs=-+|
  Terminator : Terminator
  torques : Outport
  wires:
  position/1 -> Sum1/1
  Sum1/1 -> Scope/1, PID left/1(error)
  velocity/1 -> PID left/2(velocity)
  PID left/1(torques_des) -> torques/1
  Constant/1 -> Demux1/1
  Mux1/1 -> Sum1/2
  Demux1/2 -> Mux1/2
  Demux1/4 -> Mux1/4
  theta5/1 -> Mux1/1
  Demux1/3 -> Mux1/3
  Demux1/1 -> Terminator/1

== system Control_model_10DOF_fin/Control/Inititial_Transfert/Left stance phase1/Subsystem ==
  DCM_position : Inport
  DCM_velocity : Inport  Port=2
  FK_info : Inport  Port=3
  Bus Selector : BusSelector  OutputSignals=XWcom,VWcom
  Bus Selector1 : BusSelector  OutputSignals=JRcom,JLcom,TWR,TWL,XRcom,XLcom
  Bus Selector3 : BusSelector  OutputSignals=TWR,TWL
  Bus Selector4 : BusSelector  OutputSignals=XWcom
  MATLAB Function : MATLAB Function  TreatAsAtomicUnit=on
  MATLAB Function3 : MATLAB Function  TreatAsAtomicUnit=on
  MATLAB Function5 : MATLAB Function  TreatAsAtomicUnit=on
  Scope x2 : Subsystem
  Scope x3 : Subsystem
  Scope1 : Scope
  Terminator : Terminator
  Terminator1 : Terminator
  Terminator2 : Terminator
  VRP based DCM tracking control : MATLAB Function  TreatAsAtomicUnit=on
  extrapolated CoM calcul : MATLAB Function  TreatAsAtomicUnit=on
  Torques_des : Outport  OutDataTypeStr=double  Unit=N*m
  Force_des : Outport  Port=2
  r_vrp : Outport  Port=3
  r_extrapolated_CoM : Outport  Port=4
  wires:
  DCM_position/1 -> MATLAB Function5/2(r_DCM_W), VRP based DCM tracking control/3(DCM_position)
  MATLAB Function/1(Force_des) -> Force_des/1, MATLAB Function3/1(Force_des)
  extrapolated CoM calcul/1(r_extrapolate_CoM) -> r_extrapolated_CoM/1, VRP based DCM tracking control/1(r_extrapolated_CoM)
  DCM_velocity/1 -> VRP based DCM tracking control/2(DCM_velocity)
  FK_info/1 -> Bus Selector/1, Bus Selector3/1, Bus Selector1/1, Bus Selector4/1
  VRP based DCM tracking control/1(r_vrp) -> MATLAB Function5/1(r_vrp_W)
  Bus Selector/1 -> Scope x3/1(Input), extrapolated CoM calcul/1(CoM_position)  "<XWcom>"
  Bus Selector/2 -> Scope x2/1(Input), extrapolated CoM calcul/2(CoM_velocity)  "<VWcom>"
  Bus Selector3/1 -> MATLAB Function5/3(TWR)  "<TWR>"
  Bus Selector4/1 -> MATLAB Function/2(r_CoM)  "<XWcom>"
  Bus Selector3/2 -> MATLAB Function5/4(TWL)  "<TWL>"
  MATLAB Function5/1(new_vrp_W) -> MATLAB Function/1(r_vrp), r_vrp/1
  MATLAB Function3/1(Torques_des) -> Torques_des/1
  MATLAB Function3/2(alpha) -> Scope1/1
  Bus Selector1/6 -> MATLAB Function3/7(XLcom)  "<XLcom>"
  Bus Selector1/5 -> MATLAB Function3/6(XRcom)  "<XRcom>"
  Bus Selector1/4 -> MATLAB Function3/5(TWL)  "<TWL>"
  Bus Selector1/3 -> MATLAB Function3/4(TWR)  "<TWR>"
  Bus Selector1/2 -> MATLAB Function3/3(JcomL)  "<JLcom>"
  Bus Selector1/1 -> MATLAB Function3/2(JcomR)  "<JRcom>"
  MATLAB Function5/2(new_vrp_R) -> Terminator/1
  MATLAB Function5/3(outside) -> Terminator1/1
  MATLAB Function5/4(cas) -> Terminator2/1

== system Control_model_10DOF_fin/Control/Inititial_Transfert/Right stance phase/Stance leg position_initial ==
  position : Inport  PortDimensions=4
  velocity : Inport  Port=2  PortDimensions=4
  theta4 : Inport  Port=3
  Constant : Constant  Value=jointsinitial(1:4)
  Demux : Demux
  Mux : Mux
  PID right : Subsystem
  Scope x2 : Subsystem
  Sum1 : Sum  Inputs=-+|
  Terminator : Terminator
  torques : Outport
  wires:
  PID right/1(torques_des) -> torques/1
  position/1 -> Scope x2/1(Input), Sum1/1
  Sum1/1 -> PID right/1(error)
  velocity/1 -> PID right/2(velocity)
  Constant/1 -> Demux/1
  Mux/1 -> Scope x2/2(Input1), Sum1/2
  Demux/1 -> Mux/1
  Demux/3 -> Mux/3
  theta4/1 -> Mux/4
  Demux/2 -> Mux/2
  Demux/4 -> Terminator/1

== system Control_model_10DOF_fin/Control/Inititial_Transfert/Right stance phase/Stance leg position_initial1 ==
  position : Inport  PortDimensions=4
  velocity : Inport  Port=2  PortDimensions=4
  theta5 : Inport  Port=3
  Constant : Constant  Value=jointsinitial(5:8)
  Demux1 : Demux
  Mux1 : Mux
  PID left : Subsystem
  Scope x2 : Subsystem
  Sum1 : Sum  Inputs=-+|
  Terminator : Terminator
  torques : Outport
  wires:
  position/1 -> Scope x2/1(Input), Sum1/1
  Sum1/1 -> PID left/1(error)
  velocity/1 -> PID left/2(velocity)
  PID left/1(torques_des) -> torques/1
  Constant/1 -> Demux1/1
  Mux1/1 -> Scope x2/2(Input1), Sum1/2
  Demux1/2 -> Mux1/2
  Demux1/3 -> Mux1/3
  Demux1/4 -> Mux1/4
  theta5/1 -> Mux1/1
  Demux1/1 -> Terminator/1

== system Control_model_10DOF_fin/Control/Inititial_Transfert/Right stance phase/Subsystem ==
  DCM_position : Inport
  DCM_velocity : Inport  Port=2
  FK_info : Inport  Port=3
  Bus Selector : BusSelector  OutputSignals=XWcom,VWcom
  Bus Selector1 : BusSelector  OutputSignals=JRcom,JLcom,XRcom,XLcom,TWR,TWL
  Bus Selector3 : BusSelector  OutputSignals=TWR,TWL
  Bus Selector4 : BusSelector  OutputSignals=XWcom
  MATLAB Function : MATLAB Function  TreatAsAtomicUnit=on
  MATLAB Function1 : MATLAB Function  TreatAsAtomicUnit=on
  MATLAB Function2 : MATLAB Function  TreatAsAtomicUnit=on
  Scope1 : Scope
  Terminator : Terminator
  Terminator1 : Terminator
  VRP based DCM tracking control : MATLAB Function  TreatAsAtomicUnit=on
  extrapolated CoM calcul : MATLAB Function  TreatAsAtomicUnit=on
  Torques_des : Outport  OutDataTypeStr=double  Unit=N*m
  Force_des : Outport  Port=2
  r_vrp : Outport  Port=3
  r_extrapolated_CoM : Outport  Port=4
  wires:
  Bus Selector1/1 -> MATLAB Function1/2(JcomR)  "<JRcom>"
  Bus Selector1/3 -> MATLAB Function1/4(CoM_position_R)  "<XRcom>"
  DCM_position/1 -> MATLAB Function2/2(r_DCM_W), VRP based DCM tracking control/3(DCM_position)
  Bus Selector1/4 -> MATLAB Function1/5(CoM_position_L)  "<XLcom>"
  MATLAB Function1/1(Torques_des) -> Torques_des/1
  MATLAB Function/1(Force_des) -> Force_des/1, MATLAB Function1/1(Force_des)
  Bus Selector1/2 -> MATLAB Function1/3(JcomL)  "<JLcom>"
  extrapolated CoM calcul/1(r_extrapolate_CoM) -> r_extrapolated_CoM/1, VRP based DCM tracking control/1(r_extrapolated_CoM)
  DCM_velocity/1 -> VRP based DCM tracking control/2(DCM_velocity)
  FK_info/1 -> Bus Selector/1, Bus Selector1/1, Bus Selector4/1, Bus Selector3/1
  VRP based DCM tracking control/1(r_vrp) -> MATLAB Function2/1(r_vrp_W)
  MATLAB Function1/2(alpha) -> Scope1/1
  Bus Selector/1 -> extrapolated CoM calcul/1(CoM_position)  "<XWcom>"
  Bus Selector/2 -> extrapolated CoM calcul/2(CoM_velocity)  "<VWcom>"
  Bus Selector3/1 -> MATLAB Function2/3(TWR)  "<TWR>"
  Bus Selector4/1 -> MATLAB Function/2(r_CoM)  "<XWcom>"
  MATLAB Function2/1(new_vrp_W) -> r_vrp/1, MATLAB Function/1(r_vrp)
  Bus Selector3/2 -> MATLAB Function2/4(TWL)  "<TWL>"
  Bus Selector1/5 -> MATLAB Function1/6(TWR)  "<TWR>"
  Bus Selector1/6 -> MATLAB Function1/7(TWL)  "<TWL>"
  MATLAB Function2/2(outside) -> Terminator/1
  MATLAB Function2/3(cas) -> Terminator1/1

== system Control_model_10DOF_fin/Control/Single_Support/Left Swing // Right Stance/Left Swing leg control ==
  swing_state : Inport
  actual_joint_angle : Inport  Port=2
  FK_info : Inport  Port=3
  actual_joint_velocity : Inport  Port=4
  theta7 : Inport  Port=5
  Bus Selector : BusSelector  OutputSignals=TR5,TR8,TR9,TRL,TWR
  Left : MATLAB Function  TreatAsAtomicUnit=on
  PID left : Subsystem
  Saturation : Saturate  UpperLimit=validity_angle(5:8,2)  LowerLimit=validity_angle(5:8,1)
  Scope : Scope
  Scope x1 : Subsystem
  Scope x2 : Subsystem
  Sum : Sum  Inputs=-+|
  Terminator : Terminator
  Torques_des : Outport  OutDataTypeStr=double  Unit=N*m  PortDimensions=4
  wires:
  Left/1(desired_joint_angle) -> Saturation/1
  Sum/1 -> PID left/1(error)
  actual_joint_angle/1 -> Left/8(actual_joint_angle), Scope x2/1(Input), Sum/1
  FK_info/1 -> Bus Selector/1
  actual_joint_velocity/1 -> PID left/2(velocity)
  PID left/1(torques_des) -> Torques_des/1
  swing_state/1 -> Scope x1/1(Input), Left/6(swing_state)
  Bus Selector/3 -> Left/3(TR9)  "<TR9>"
  Bus Selector/4 -> Left/4(TRL)  "<TRL>"
  Bus Selector/1 -> Left/1(TR5)  "<TR5>"
  Saturation/1 -> Sum/2, Scope x2/2(Input1)
  Bus Selector/2 -> Left/2(TR8)  "<TR8>"
  Bus Selector/5 -> Left/5(TWR)  "<TWR>"
  Left/3(cas) -> Scope/1
  theta7/1 -> Left/7(desired_knee_angle)
  Left/2(ok) -> Terminator/1

== system Control_model_10DOF_fin/Control/Single_Support/Left Swing // Right Stance/Martijn Step adjustement ==
  FK_info : Inport
  R_or_L : Inport  Port=2
  Bus Selector : BusSelector  OutputSignals=XWcom,VWcom
  Constant1 : Constant  Value=time_swing
  Terminator : Terminator
  xCoM pred : Subsystem
  StepPos : Outport
  wires:
  Constant1/1 -> xCoM pred/1(T)
  R_or_L/1 -> xCoM pred/4(R_or_L)
  FK_info/1 -> Bus Selector/1
  Bus Selector/2 -> xCoM pred/3(Vcom)  "<VWcom>"
  Bus Selector/1 -> xCoM pred/2(Xcom)  "<XWcom>"
  xCoM pred/1(StepPos) -> StepPos/1
  xCoM pred/2(xCoMpred) -> Terminator/1

== system Control_model_10DOF_fin/Control/Single_Support/Left Swing // Right Stance/Right Stance leg control ==
  DCM_position : Inport
  DCM_velocity : Inport  Port=2
  FK_info : Inport  Port=3
  Bus Selector : BusSelector  OutputSignals=XWcom,VWcom
  Bus Selector1 : BusSelector  OutputSignals=JRcom,TWR
  Bus Selector3 : BusSelector  OutputSignals=TWR
  Bus Selector4 : BusSelector  OutputSignals=XWcom
  DCM calcul : MATLAB Function  TreatAsAtomicUnit=on
  MATLAB Function : MATLAB Function  TreatAsAtomicUnit=on
  MATLAB Function1 : MATLAB Function  TreatAsAtomicUnit=on
  MATLAB Function2 : MATLAB Function  TreatAsAtomicUnit=on
  MATLAB Function5 : MATLAB Function  TreatAsAtomicUnit=on
  Terminator : Terminator
  Terminator1 : Terminator
  VRP based DCM tracking control : MATLAB Function  TreatAsAtomicUnit=on
  Torques_des : Outport  OutDataTypeStr=double  Unit=N*m
  Force_des : Outport  Port=2
  r_vrp : Outport  Port=3
  r_extrapolated_CoM : Outport  Port=4
  wires:
  Bus Selector1/1 -> MATLAB Function1/2(JcomR)  "<JRcom>"
  MATLAB Function1/1(Torques_des) -> Torques_des/1
  DCM_position/1 -> VRP based DCM tracking control/3(DCM_position)
  MATLAB Function/1(Force_des) -> MATLAB Function1/1(Force_des_W)
  DCM_velocity/1 -> VRP based DCM tracking control/2(DCM_velocity)
  DCM calcul/1(r_extrapolated_CoM) -> VRP based DCM tracking control/1(r_extrapolated_CoM), r_extrapolated_CoM/1
  FK_info/1 -> Bus Selector1/1, Bus Selector4/1, Bus Selector3/1, Bus Selector/1
  Bus Selector/1 -> DCM calcul/1(CoM_position)  "<XWcom>"
  Bus Selector4/1 -> MATLAB Function2/2(r_CoM), MATLAB Function/2(r_CoM)  "<XWcom>"
  Bus Selector/2 -> DCM calcul/2(CoM_velocity)  "<VWcom>"
  Bus Selector3/1 -> MATLAB Function2/3(TWR), MATLAB Function5/2(TWR)  "<TWR>"
  VRP based DCM tracking control/1(r_vrp) -> MATLAB Function2/1(r_vrp), MATLAB Function5/1(r_vrp_W)
  MATLAB Function5/1(new_vrp_W) -> r_vrp/1, MATLAB Function/1(r_vrp)
  Bus Selector1/2 -> MATLAB Function1/3(TWR)  "<TWR>"
  MATLAB Function2/1(Force_des) -> Force_des/1
  MATLAB Function5/2(outside) -> Terminator/1
  MATLAB Function5/3(cas) -> Terminator1/1

== system Control_model_10DOF_fin/Control/Single_Support/Left Swing // Right Stance/Scope x1 ==
  Input : Inport
  Demux : Demux  Outputs=3
  Scope1 : Scope
  Scope2 : Scope
  Scope3 : Scope
  wires:
  Input/1 -> Demux/1
  Demux/2 -> Scope1/1
  Demux/3 -> Scope2/1
  Demux/1 -> Scope3/1
